simulink model "Task3_Integral_MRAC"  (R2024b)
settings: Solver=ode45  StartTime=0.0  StopTime=80  MaxStep=0.01  RelTol=1e-7  AbsTol=1e-9
settings Model: Creator=LAPTOPASADI  LastModifiedBy=LAPTOPASADI
settings DataIOCC: SaveOutput=off  SignalLogging=off  SaveTime=off  ReturnWorkspaceOutputs=off

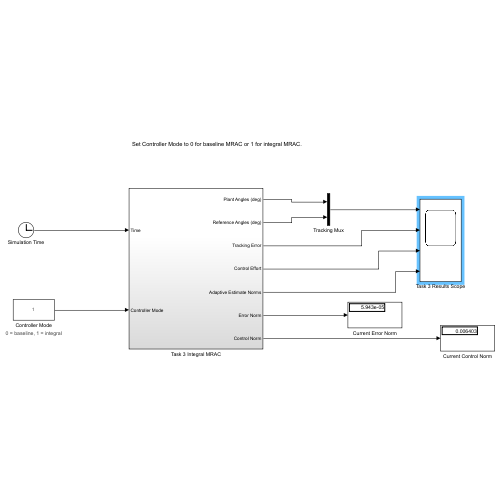
[thumbnail: Simulink's stored preview of the top-level diagram]
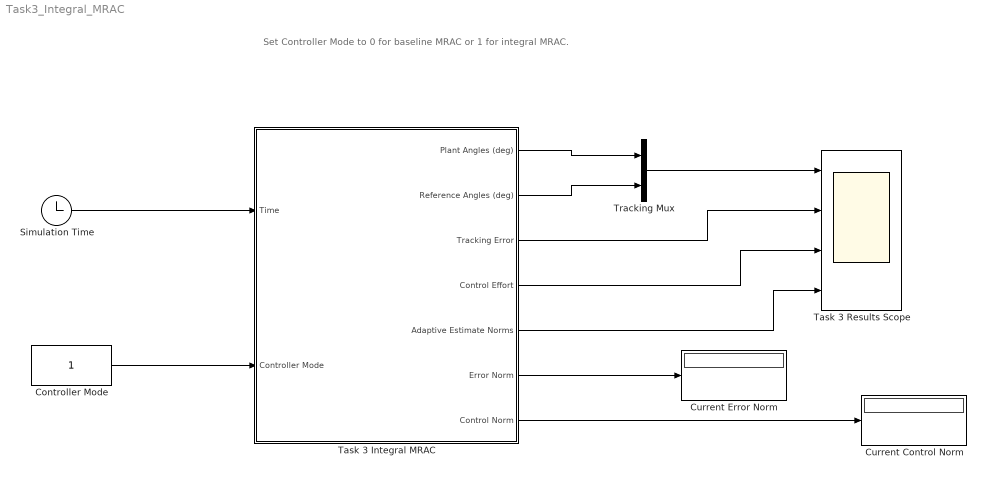
== system Task3_Integral_MRAC ==
  note: Set Controller Mode to 0 for baseline MRAC or 1 for integral MRAC.
  Controller Mode : Constant
      settings: AttributesFormatString=0 = baseline, 1 = integral
  Current Control Norm : Display
  Current Error Norm : Display
  Simulation Time : Clock
  Task 3 Integral MRAC : Subsystem
  Task 3 Results Scope : Scope  NumInputPorts=4
  Tracking Mux : Mux  Inputs=2
  wires:
  Simulation Time/1 -> Task 3 Integral MRAC/1(Time)
  Controller Mode/1 -> Task 3 Integral MRAC/2(Controller Mode)
  Task 3 Integral MRAC/1(Plant Angles (deg)) -> Tracking Mux/1
  Task 3 Integral MRAC/2(Reference Angles (deg)) -> Tracking Mux/2
  Tracking Mux/1 -> Task 3 Results Scope/1
  Task 3 Integral MRAC/3(Tracking Error) -> Task 3 Results Scope/2
  Task 3 Integral MRAC/4(Control Effort) -> Task 3 Results Scope/3
  Task 3 Integral MRAC/5(Adaptive Estimate Norms) -> Task 3 Results Scope/4
  Task 3 Integral MRAC/6(Error Norm) -> Current Error Norm/1
  Task 3 Integral MRAC/7(Control Norm) -> Current Control Norm/1

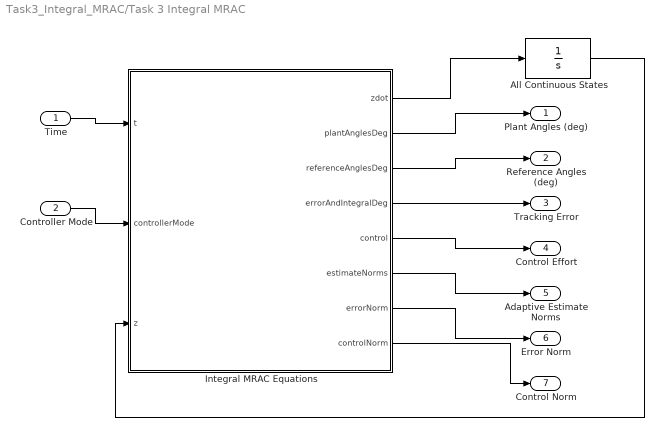
== system Task3_Integral_MRAC/Task 3 Integral MRAC ==
  Time : Inport
  Controller Mode : Inport  Port=2
  All Continuous States : Integrator  InitialCondition=[0;0;0;0;0;0;0;0;0;0;0;0;0;0;0;0;-0.66823529411764704;0;0;-0.66823529411764704;0;-0.093784508916032808;0;-0.084095775670305087;-0.093784508916032808;0;-0.084095775670305087;-0.020546127010358625;0;0.38386217602841338;-0.020546127010358625;0;0.38386217602841338;0;0;0;0;0;0;0;0;0;0;0.66823529411764704;0;0.093784508916032808;0;0.084095775670305087;0.020546127010358625;0;-0.38386217602841338;0;0.15647058823529411;0;0;-0.0016705882352941175;0;-0.018538798274099509;0;-0.011825968453636653;-0.00023446127229008202;0;-0.00021023943917576274;-0.0040614437113499612;0;0.053980618503995631;-5.1365317525896568e-05;0;0.00095965544007103345]
  Integral MRAC Equations : MATLAB Function  TreatAsAtomicUnit=on
  Plant Angles (deg) : Outport
  Reference Angles (deg) : Outport  Port=2
  Tracking Error : Outport  Port=3
  Control Effort : Outport  Port=4
  Adaptive Estimate Norms : Outport  Port=5
  Error Norm : Outport  Port=6
  Control Norm : Outport  Port=7
  wires:
  Time/1 -> Integral MRAC Equations/1(t)
  Controller Mode/1 -> Integral MRAC Equations/2(controllerMode)
  All Continuous States/1 -> Integral MRAC Equations/3(z)
  Integral MRAC Equations/1(zdot) -> All Continuous States/1
  Integral MRAC Equations/2(plantAnglesDeg) -> Plant Angles (deg)/1
  Integral MRAC Equations/3(referenceAnglesDeg) -> Reference Angles (deg)/1
  Integral MRAC Equations/4(errorAndIntegralDeg) -> Tracking Error/1
  Integral MRAC Equations/5(control) -> Control Effort/1
  Integral MRAC Equations/6(estimateNorms) -> Adaptive Estimate Norms/1
  Integral MRAC Equations/7(errorNorm) -> Error Norm/1
  Integral MRAC Equations/8(controlNorm) -> Control Norm/1

== matlab function Task3_Integral_MRAC/Task 3 Integral MRAC/Integral MRAC Equations ==
  data: t input; zdot output; controllerMode input; z input; plantAnglesDeg output; referenceAnglesDeg output; errorAndIntegralDeg output; control output; estimateNorms output; errorNorm output; controlNorm output
function [zdot,plantAnglesDeg,referenceAnglesDeg,errorAndIntegralDeg,control,estimateNorms,errorNorm,controlNorm] = integralMRAC(t,controllerMode,z)
%#codegen
% Standalone Task 3 equations. Mode 0 is baseline; mode 1 adds integral action.

x = z(1:6);
xm = z(7:12);
eI = z(13:15);
KxHat = reshape(z(16:33),6,3);
KiHat = reshape(z(34:42),3,3);
KrHat = reshape(z(43:51),3,3);
ThetaHat = reshape(z(52:69),6,3);

dOverB = 1.2e-6/3.13e-5;
G = [0,0.175/0.0043,dOverB/0.0043; ...
     0.085/0.0142,0,0; ...
     0,dOverB/0.0176,-0.175/0.0176];
aP = (0.0142-0.0176)/0.0043;
aQ = (0.0176-0.0043)/0.0142;
aR = (0.0043-0.0142)/0.0176;
Htrue = [aP,0,0,-0.01,0,0; ...
         0,aQ,0,0,-0.01,0; ...
         0,0,aR,0,0,-0.01];
B = [zeros(3,3);G];

p = x(4);
q = x(5);
rBody = x(6);
Phi = [q*rBody;p*rBody;p*q;p;q;rBody];
reference = zeros(3,1);
error = x-xm;

if controllerMode < 0.5
    control = KxHat.'*x + KrHat.'*reference - ThetaHat.'*Phi;
else
    control = KxHat.'*x + KiHat.'*eI + KrHat.'*reference - ThetaHat.'*Phi;
end

inputDisturbance = zeros(3,1);
if t >= 20
    inputDisturbance = [0.004;-0.003;0.004];
end
xdot = [x(4:6);G*(control+inputDisturbance)+Htrue*Phi];
xmdot = [xm(4:6);-4*xm(1:3)-4*xm(4:6)+4*reference];
eIdot = error(1:3);

P = [1.125*eye(3),0.125*eye(3); ...
     0.125*eye(3),0.15625*eye(3)];
if controllerMode < 0.5
    signal = error.'*P*B;
    KxHatDot = -50*x*signal;
    KiHatDot = zeros(3,3);
    KrHatDot = -50*reference*signal;
    ThetaHatDot = 50*Phi*signal;
else
    Pbar = [2.749999999999996 0 0 0.49999999999999767 0 0 1.4999999999999973 0 0;0 2.749999999999996 0 0 0.49999999999999767 0 0 1.4999999999999973 0;0 0 2.749999999999996 0 0 0.49999999999999767 0 0 1.4999999999999973;0.49999999999999767 0 0 0.24999999999999903 0 0 0.24999999999999867 0 0;0 0.49999999999999767 0 0 0.24999999999999903 0 0 0.24999999999999867 0;0 0 0.49999999999999767 0 0 0.24999999999999897 0 0 0.24999999999999867;1.4999999999999973 0 0 0.24999999999999867 0 0 1.999999999999998 0 0;0 1.4999999999999973 0 0 0.24999999999999867 0 0 1.999999999999998 0;0 0 1.4999999999999973 0 0 0.24999999999999867 0 0 1.9999999999999978];
    Bbar = [B;zeros(3,3)];
    GammaBar = [50 0 0 0 0 0 0 0 0;0 50 0 0 0 0 0 0 0;0 0 50 0 0 0 0 0 0;0 0 0 50 0 0 0 0 0;0 0 0 0 50 0 0 0 0;0 0 0 0 0 50 0 0 0;0 0 0 0 0 0 25 0 0;0 0 0 0 0 0 0 25 0;0 0 0 0 0 0 0 0 25];
    signal = [error;eI].'*Pbar*Bbar;
    KbarHatDot = -GammaBar*[x;eI]*signal;
    KxHatDot = KbarHatDot(1:6,:);
    KiHatDot = KbarHatDot(7:9,:);
    KrHatDot = -50*reference*signal;
    ThetaHatDot = 50*Phi*signal;
end

zdot = [xdot;xmdot;eIdot;KxHatDot(:);KiHatDot(:);KrHatDot(:);ThetaHatDot(:)];
plantAnglesDeg = (180/pi)*x(1:3);
referenceAnglesDeg = (180/pi)*xm(1:3);
errorAndIntegralDeg = (180/pi)*[error(1:3);eI];
estimateNorms = [sqrt(sum(KxHat(:).^2)); ...
                 sqrt(sum(KiHat(:).^2)); ...
                 sqrt(sum(KrHat(:).^2)); ...
                 sqrt(sum(ThetaHat(:).^2))];
errorNorm = sqrt(sum(error(1:3).^2));
controlNorm = sqrt(sum(control.^2));
end
